simulink model "afr_2016b"  (R2016b)
settings: Solver=VariableStepAuto  StartTime=0.0  StopTime=40  RelTol=1e-3
InitFcn:
  | clear all;
StopFcn:
  | plots
settings Model: Creator=Captain  LastModifiedBy=Ruslan.Sevostianov
settings SFSimCC: SimUseLocalCustomCode=on
settings RTWCC: RTWUseLocalCustomCode=on

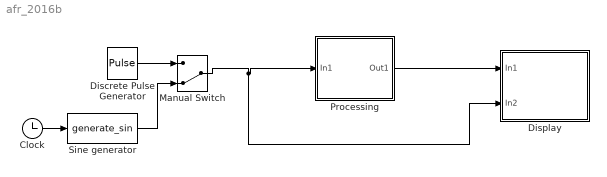
== system afr_2016b ==
  Clock : Clock
  Discrete Pulse Generator : DiscretePulseGenerator  Period=100  PhaseDelay=2  SampleTime=0.005
  Display : Subsystem
  Manual Switch : ManualSwitch  CurrentSetting=0
  Processing : Subsystem
  Sine generator : MATLABFcn  MATLABFcn=generate_sin
  wires:
  Processing/1(Out1) -> Display/1(In1)
  Discrete Pulse Generator/1 -> Manual Switch/1
  Manual Switch/1 -> Display/2(In2), Processing/1(In1)
  Sine generator/1 -> Manual Switch/2
  Clock/1 -> Sine generator/1

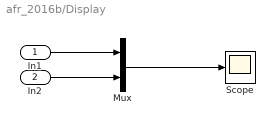
== system afr_2016b/Display ==
  In1 : Inport
  In2 : Inport  Port=2
  Mux : Mux  Inputs=2
  Scope : Scope
  wires:
  Mux/1 -> Scope/1
  In2/1 -> Mux/2
  In1/1 -> Mux/1

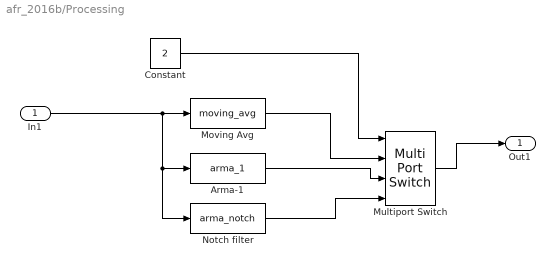
== system afr_2016b/Processing ==
  In1 : Inport
  Arma-1 : MATLABFcn  MATLABFcn=arma_1
  Constant : Constant  Value=2
  Moving Avg : MATLABFcn  MATLABFcn=moving_avg
  Multiport Switch : MultiPortSwitch
  Notch filter : MATLABFcn  MATLABFcn=arma_notch
  Out1 : Outport
  wires:
  In1/1 -> Notch filter/1, Arma-1/1, Moving Avg/1
  Moving Avg/1 -> Multiport Switch/2
  Notch filter/1 -> Multiport Switch/4
  Multiport Switch/1 -> Out1/1
  Arma-1/1 -> Multiport Switch/3
  Constant/1 -> Multiport Switch/1
